simulink model "twowheeledrobot_temp"  (R2023b)
settings: Solver=ode4  StartTime=0  StopTime=100  FixedStep=1e-2  RelTol=1e-3  AbsTol=1e-6
settings Model: Creator=jerome  LastModifiedBy=jerome
settings SolverCC: AutoScaleAbsTol=off  AlgebraicLoopSolver=TrustRegion
settings DataIOCC: SaveFormat=Array  SignalLoggingSaveFormat=ModelDataLogs  ReturnWorkspaceOutputs=off
settings OptimizationCC: BlockReduction=off  BooleanDataType=off  ExpressionDepthLimit=2147483647  InitFltsAndDblsToZero=on  LifeSpan=inf
settings DebuggingCC: SaveWithParameterizedLinksMsg=none  UnderspecifiedInitializationDetection=Classic  MergeDetectMultiDrivingBlocksExec=none  SignalResolutionControl=TryResolveAllWithWarning  MultiTaskDSMMsg=warning  MultiTaskCondExecSysMsg=none  FcnCallInpInsideContextMsg=warning  UnconnectedInputMsg=warning  UnconnectedOutputMsg=warning  UnconnectedLineMsg=warning  StateNameClashWarn=warning  SFUnexpectedBacktrackingDiag=warning  SFNoUnconditionalDefaultTransitionDiag=warning  SFExecutionAtInitializationDiag=none  ArithmeticOperatorsInVariantConditions=warning
settings HardwareCC: ProdBitPerPointer=32  ProdBitPerSizeT=32  ProdBitPerPtrDiffT=32  ProdLargestAtomicFloat=None  ProdIntDivRoundTo=Undefined  ProdEndianess=Unspecified  ProdWordSize=32  ProdHWDeviceType=32-bit Generic  TargetUnknown=on
settings ModelReferenceCC: EnableRefExpFcnMdlSchedulingChecks=on  PropagateSignalLabelsOutOfModel=off
settings SFSimCC: SimUseLocalCustomCode=off  CustomCodeUndefinedFunction=UseInterfaceOnly
settings RTWCC: RTWUseLocalCustomCode=off  DLArmComputeVersion=19.05
settings CodeAppCC: StateflowObjectComments=on
settings GRTTargetCC: TargetFcnLib=ansi_tfl_tmw.mat  TargetLangStandard=C89/C90 (ANSI)  ModelReferenceCompliant=off  CombineOutputUpdateFcns=off  MatFileLogging=off  GRTInterface=on
settings ConfigComp: CovMetricSettings=dw  CovSaveCumulativeToWorkspaceVar=on  CovSaveSingleToWorkspaceVar=on  CovExternalEMLEnable=off

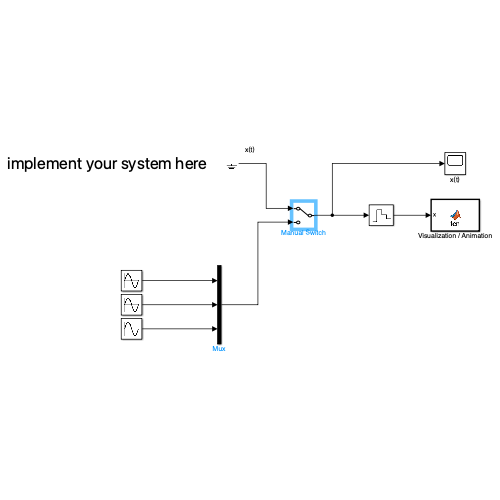
[thumbnail: Simulink's stored preview of the top-level diagram]
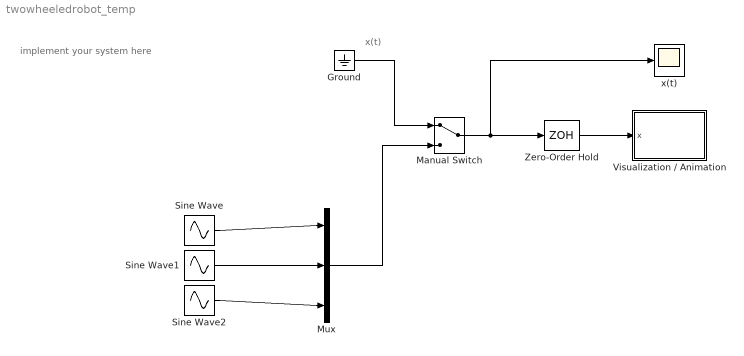
== system twowheeledrobot_temp ==
  note: implement your system here
  note: x(t)
  Ground : Ground
  Manual Switch : ManualSwitch
  Mux : Mux  Inputs=3
  Sine Wave : Sin  Amplitude=2  Bias=1  SampleTime=0
  Sine Wave1 : Sin  Amplitude=2  Bias=3  SampleTime=0
  Sine Wave2 : Sin  Amplitude=pi/4  SampleTime=0
  Visualization / Animation : MATLAB Function  TreatAsAtomicUnit=on
  Zero-Order Hold : ZeroOrderHold  SampleTime=0.1
  x(t) : Scope
  wires:
  Zero-Order Hold/1 -> Visualization / Animation/1(x)
  Manual Switch/1 -> Zero-Order Hold/1, x(t)/1
  Ground/1 -> Manual Switch/1
  Mux/1 -> Manual Switch/2
  Sine Wave/1 -> Mux/1
  Sine Wave2/1 -> Mux/3
  Sine Wave1/1 -> Mux/2

== matlab function twowheeledrobot_temp/Visualization // Animation ==
  data: x input
function fcn(x)


% body
    Ybody = [ -0.2 ; -0.2 ; 0.2 ; 0.2 ];
    Xbody = [ -0.15 ; 0.15 ; 0.15 ; -0.15 ]; 

% front
    Yfront = [ -0.2 ; -0.1 ; 0.1 ; 0.2 ];
    Xfront = [ 0.15 ; 0.2 ; 0.2 ; 0.15 ];
    
% wheel model
    Yw = [ -0.02 ; -0.02 ; 0.02 ; 0.02 ];
    Xw = [ -0.13 ; 0.13 ; 0.13 ; -0.13 ];
    
% left wheel
    Ywl = Yw + 0.21;
    Xwl = Xw;
    
% right wheel    
    Ywr = Yw - 0.21;
    Xwr = Xw;

% calculate graphical position of 2-wheel robot
      [PosXbody,PosYbody] = rot(Xbody,Ybody,x(3));
      PosXbody = PosXbody + x(1);
      PosYbody = PosYbody + x(2);

      [PosXwl,PosYwl] = rot(Xwl,Ywl,x(3));
      PosXwl = PosXwl + x(1);
      PosYwl = PosYwl + x(2);

      [PosXwr,PosYwr] = rot(Xwr,Ywr,x(3));
      PosXwr = PosXwr + x(1);
      PosYwr = PosYwr + x(2);

      [PosXfront,PosYfront] = rot(Xfront,Yfront,x(3));
      PosXfront = PosXfront + x(1);
      PosYfront = PosYfront + x(2);


% to be able to use 'fill' even though the function is not supported for code generation
% see https://se.mathworks.com/help/simulink/slref/coder.extrinsic.html
coder.extrinsic('fill'); 

% draw the body of the 2-wheel robot with the propser position and orientation
fill(PosXbody,PosYbody,'r');

hold on
% draw the rest of the robot
fill(PosXwl,PosYwl,'b');
fill(PosXwr,PosYwr,'b');
fill(PosXfront,PosYfront,'g');

hold off

axis([-1 6 -1 6]);
title('The 2-wheel robot', 'FontSize',20);
axis square;
grid on;

drawnow;



% function "rot" that rotates a graphical object
function [PosX,PosY] = rot(X,Y,angle)

dim = size(X,1);
PosX = zeros(dim,1);
PosY = zeros(dim,1);

Mrot = [ cos(angle) -sin(angle)  ;
         sin(angle)  cos(angle) ]; 

for i=1:dim
    Pos_i = Mrot * [ X(i,1) ; Y(i,1) ];
    PosX(i,1) = Pos_i(1,1);
    PosY(i,1) = Pos_i(2,1);
end
